simulink model "POMS_model_expanded"  (Simulink 7.9)
settings: Solver=VariableStepDiscrete  StartTime=0.0  StopTime=100.0  RelTol=1e-3
(part 2 of 2)

== system POMS_model_expanded/Depot_2/Storage_Subsystem/<<DELIVER>>Deliver_Stocked_Product/Deliver_Stocked_Product_CONTROL ==
  Calculate_Inventory_C : MATLAB Function  TreatAsAtomicUnit=on
  Combine_Consumption_Inventory : EntityCombiner  NumberInputPorts=2
  Consumption_Attributes : GetAttribute  AttributeName=Component|Consumption_Quantity|Net_Inventory|Inventory_Position  AttributeMissing=Error|Error|Error|Error  AttributeDefaultValue=1|1|1|1  AttributeTreatAsVector=1|1|1|1  AttributeSendTiming=After entity departure|After entity departure|After entity departure|After entity departure  EvaluatedDefaultAttributeValue={[];[];[];[]}
      settings: OutputPortMap=o1,o2,o3,o4
  Consumption_Server : SingleServer  ServiceTime=0
  Consumption_Sink : EntitySink
  Replicate : Replicate  NumberOutputPorts=2
  Return_Inventory : EntitySplitter  NumberOutputPorts=2
  Set_Inventory_Level : SetAttribute  AttributeName=Net_Inventory|Inventory_Position  AttributeFrom=Signal port|Signal port  AttributeValue=1|1  AttributeTreatAsVector=1|1  EvaluatedAttributeValue={[];[]}
      settings: InputPortMap=u0,u1
  Inventory_IN : PMIOPort  Port=1  Side=Left
  Consumption_Signal_IN : PMIOPort  Port=2  Side=Left
  Consumption_Signal_OUT : PMIOPort  Port=3  Side=Right
  Inventory_OUT : PMIOPort  Port=4  Side=Right
  wires:
  Calculate_Inventory_C/2(out_Inventory_Position) -> Set_Inventory_Level/2
  Consumption_Attributes/4 -> Calculate_Inventory_C/2(Inventory_Position)
  Consumption_Attributes/2 -> Calculate_Inventory_C/4(Consumption_Quantity)
  Consumption_Attributes/3 -> Calculate_Inventory_C/1(Net_Inventory)
  Calculate_Inventory_C/1(out_Net_Inventory) -> Set_Inventory_Level/1
  Consumption_Attributes/1 -> Calculate_Inventory_C/3(Component)
  connections:
  Consumption_Signal_IN/RConn1 -- Replicate/LConn1
  Inventory_OUT/RConn1 -- Return_Inventory/RConn1
  Set_Inventory_Level/RConn1 -- Return_Inventory/LConn1
  Replicate/RConn2 -- Consumption_Signal_OUT/RConn1
  Return_Inventory/RConn2 -- Consumption_Sink/LConn1
  Consumption_Server/RConn1 -- Set_Inventory_Level/LConn1
  Consumption_Attributes/RConn1 -- Consumption_Server/LConn1
  Combine_Consumption_Inventory/RConn1 -- Consumption_Attributes/LConn1
  Replicate/RConn1 -- Combine_Consumption_Inventory/LConn2
  Inventory_IN/RConn1 -- Combine_Consumption_Inventory/LConn1

== system POMS_model_expanded/Depot_2/Storage_Subsystem/<<DELIVER>>Deliver_Stocked_Product/sD1.10_Pack_Order_PLANT ==
  Entity Departure Function-Call Generator : EntityDepartureFunctionCallGenerator
  Event-Based Entity Generator : EventBasedEntityGenerator  GenerateEntitiesUpon=Function call from port fcn
  Get_Order_Attribute : GetAttribute  AttributeName=Component|Order_Quantity|Customer  AttributeMissing=Error|Error|Error  AttributeDefaultValue=1|1|1  AttributeTreatAsVector=1|1|1  AttributeSendTiming=After entity departure|After entity departure|After entity departure  EvaluatedDefaultAttributeValue={[];[];[]}
      settings: OutputPortMap=o1,o2,o3
  Order_Sink : EntitySink
  Set_Shipment_Attributes : SetAttribute  AttributeName=Component|Shipment_Quantity|Customer  AttributeFrom=Signal port|Signal port|Signal port  AttributeValue=1|1|1  AttributeTreatAsVector=1|1|1  EvaluatedAttributeValue={[];[];[]}
      settings: InputPortMap=u0,u1,u2
  sD1.10_Queue : FIFOQueue
  sD1.10_Server : NServer  NumberOfServers=inf  ServiceTime=0
  Order_IN : PMIOPort  Port=1  Side=Left
  Shipment_OUT : PMIOPort  Port=2  Side=Right
  wires:
  Get_Order_Attribute/3 -> Set_Shipment_Attributes/3
  Get_Order_Attribute/1 -> Set_Shipment_Attributes/1
  Get_Order_Attribute/2 -> Set_Shipment_Attributes/2
  Entity Departure Function-Call Generator/1 -> Event-Based Entity Generator/1
  connections:
  Get_Order_Attribute/RConn1 -- Entity Departure Function-Call Generator/LConn1
  sD1.10_Server/RConn1 -- Get_Order_Attribute/LConn1
  Order_Sink/LConn1 -- Entity Departure Function-Call Generator/RConn1
  Set_Shipment_Attributes/RConn1 -- Shipment_OUT/RConn1
  Event-Based Entity Generator/RConn1 -- Set_Shipment_Attributes/LConn1
  Order_IN/RConn1 -- sD1.10_Queue/LConn1
  sD1.10_Queue/RConn1 -- sD1.10_Server/LConn1

== system POMS_model_expanded/Depot_2/Storage_Subsystem/<<DELIVER>>Deliver_Stocked_Product/sD1.11_Load_Order_PLANT ==
  sD1.11_Queue : FIFOQueue
  sD1.11_Server : NServer  NumberOfServers=inf  ServiceTime=0
  Shipment_IN : PMIOPort  Port=1  Side=Left
  Shipment_OUT : PMIOPort  Port=2  Side=Right
  connections:
  Shipment_OUT/RConn1 -- sD1.11_Server/RConn1
  Shipment_IN/RConn1 -- sD1.11_Queue/LConn1
  sD1.11_Queue/RConn1 -- sD1.11_Server/LConn1

== system POMS_model_expanded/Depot_2/Storage_Subsystem/<<DELIVER>>Deliver_Stocked_Product/sD1.2_Receive_Order_PLANT ==
  sD1.2_Queue : FIFOQueue
  sD1.2_Server : NServer  NumberOfServers=inf  ServiceTime=0
  Order_IN : PMIOPort  Port=1  Side=Left
  Order_OUT : PMIOPort  Port=2  Side=Right
  connections:
  Order_OUT/RConn1 -- sD1.2_Server/RConn1
  Order_IN/RConn1 -- sD1.2_Queue/LConn1
  sD1.2_Queue/RConn1 -- sD1.2_Server/LConn1

== system POMS_model_expanded/Depot_2/Storage_Subsystem/<<DELIVER>>Deliver_Stocked_Product/sD1.4_Consolidate_Orders_PLANT ==
  sD1.4_Queue : FIFOQueue
  sD1.4_Server : NServer  NumberOfServers=inf  ServiceTime=0
  Order_IN : PMIOPort  Port=1  Side=Left
  Order_OUT : PMIOPort  Port=2  Side=Right
  connections:
  Order_OUT/RConn1 -- sD1.4_Server/RConn1
  Order_IN/RConn1 -- sD1.4_Queue/LConn1
  sD1.4_Queue/RConn1 -- sD1.4_Server/LConn1

== system POMS_model_expanded/Depot_2/Storage_Subsystem/<<DELIVER>>Deliver_Stocked_Product/sD1.9_Pick_Order_PLANT ==
  Generate_Consumption_Signal : Subsystem
  sD1.9_Queue : FIFOQueue
  sD1.9_Server : NServer  NumberOfServers=inf  ServiceTime=0
  Order_IN : PMIOPort  Port=1  Side=Left
  Consumption_Signal : PMIOPort  Port=2  Side=Right
  Order_OUT : PMIOPort  Port=3  Side=Right
  connections:
  Generate_Consumption_Signal/RConn2 -- Consumption_Signal/RConn1
  Generate_Consumption_Signal/RConn1 -- Order_OUT/RConn1
  sD1.9_Server/RConn1 -- Generate_Consumption_Signal/LConn1
  Order_IN/RConn1 -- sD1.9_Queue/LConn1
  sD1.9_Queue/RConn1 -- sD1.9_Server/LConn1

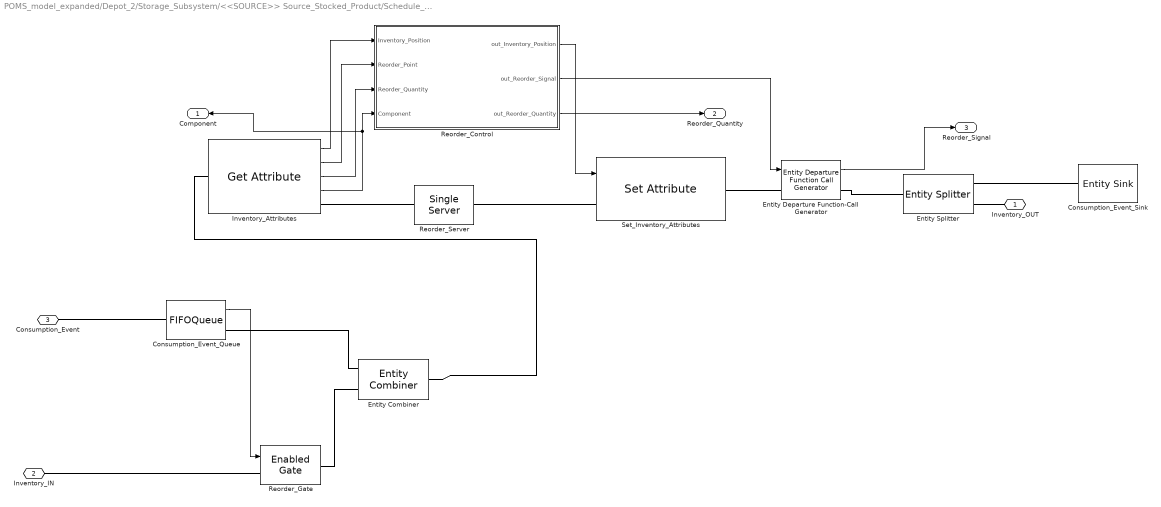
== system POMS_model_expanded/Depot_2/Storage_Subsystem/<<SOURCE>> Source_Stocked_Product/Schedule_Product_Deliveries_CONTROL ==
  Consumption_Event_Queue : FIFOQueue  StatNumberInBlock=on
      settings: OutputPortMap=o1
  Consumption_Event_Sink : EntitySink
  Entity Combiner : EntityCombiner  NumberInputPorts=2
  Entity Departure Function-Call Generator : EntityDepartureFunctionCallGenerator  EnableE1Port=on
  Entity Splitter : EntitySplitter  NumberOutputPorts=2
  Inventory_Attributes : GetAttribute  AttributeName=Inventory_Position|Reorder_Point|Reorder_Quantity|Component  AttributeMissing=Error|Error|Error|Error  AttributeDefaultValue=1|1|1|1  AttributeTreatAsVector=1|1|1|1  AttributeSendTiming=After entity departure|After entity departure|After entity departure|After entity departure  EvaluatedDefaultAttributeValue={[];[];[];[]}
      settings: OutputPortMap=o1,o2,o3,o4
  Reorder_Control : MATLAB Function  TreatAsAtomicUnit=on
  Reorder_Gate : EnabledGate
  Reorder_Server : SingleServer  ServiceTime=0
  Set_Inventory_Attributes : SetAttribute  AttributeName=Inventory_Position  AttributeFrom=Signal port  EvaluatedAttributeValue={[]}
  Inventory_OUT : PMIOPort  Port=1  Side=Right
  Inventory_IN : PMIOPort  Port=2  Side=Left
  Consumption_Event : PMIOPort  Port=3  Side=Left
  Component : Outport
  Reorder_Quantity : Outport  Port=2
  Reorder_Signal : Outport  Port=3
  wires:
  Entity Departure Function-Call Generator/1 -> Reorder_Signal/1
  Reorder_Control/3(out_Reorder_Quantity) -> Reorder_Quantity/1
  Consumption_Event_Queue/1 -> Reorder_Gate/1
  Reorder_Control/2(out_Reorder_Signal) -> Entity Departure Function-Call Generator/1
  Inventory_Attributes/4 -> Component/1, Reorder_Control/4(Component)
  Reorder_Control/1(out_Inventory_Position) -> Set_Inventory_Attributes/1
  Inventory_Attributes/3 -> Reorder_Control/3(Reorder_Quantity)
  Inventory_Attributes/2 -> Reorder_Control/2(Reorder_Point)
  Inventory_Attributes/1 -> Reorder_Control/1(Inventory_Position)
  connections:
  Entity Departure Function-Call Generator/RConn1 -- Entity Splitter/LConn1
  Set_Inventory_Attributes/RConn1 -- Entity Departure Function-Call Generator/LConn1
  Reorder_Server/RConn1 -- Set_Inventory_Attributes/LConn1
  Inventory_IN/RConn1 -- Reorder_Gate/LConn1
  Inventory_Attributes/RConn1 -- Reorder_Server/LConn1
  Inventory_OUT/RConn1 -- Entity Splitter/RConn2
  Entity Combiner/RConn1 -- Inventory_Attributes/LConn1
  Reorder_Gate/RConn1 -- Entity Combiner/LConn2
  Entity Splitter/RConn1 -- Consumption_Event_Sink/LConn1
  Consumption_Event_Queue/RConn1 -- Entity Combiner/LConn1
  Consumption_Event/RConn1 -- Consumption_Event_Queue/LConn1

== system POMS_model_expanded/Depot_2/Storage_Subsystem/<<SOURCE>> Source_Stocked_Product/Transfer_Product_CONTROL ==
  Calculate_Inventory : MATLAB Function  TreatAsAtomicUnit=on
  Combine_Inventory_and_Availability : EntityCombiner  NumberInputPorts=2
  FIFO Queue : FIFOQueue
  Inventory_Availability_Attributes : GetAttribute  AttributeName=Component|Shipment_Quantity|Net_Inventory  AttributeMissing=Error|Error|Error  AttributeDefaultValue=1|1|1  AttributeTreatAsVector=1|1|1  AttributeSendTiming=After entity departure|After entity departure|After entity departure  EvaluatedDefaultAttributeValue={[];[];[]}
      settings: OutputPortMap=o1,o2,o3
  Inventory_Availability_Sink : EntitySink
  Return_Inventory : EntitySplitter  NumberOutputPorts=2
  Server : SingleServer  ServiceTime=0
  Set_Inventory_Level : SetAttribute  AttributeName=Net_Inventory  AttributeFrom=Signal port  EvaluatedAttributeValue={[]}
  Inventory_OUT : PMIOPort  Port=1  Side=Right
  Inventory_IN : PMIOPort  Port=2  Side=Left
  Inventory_Availability_Signal : PMIOPort  Port=3  Side=Left
  wires:
  Inventory_Availability_Attributes/2 -> Calculate_Inventory/3(Shipment_Quantity)
  Inventory_Availability_Attributes/3 -> Calculate_Inventory/1(Net_Inventory)
  Calculate_Inventory/1(out_Inventory) -> Set_Inventory_Level/1
  Inventory_Availability_Attributes/1 -> Calculate_Inventory/2(Component)
  connections:
  Inventory_IN/RConn1 -- Combine_Inventory_and_Availability/LConn1
  FIFO Queue/RConn1 -- Combine_Inventory_and_Availability/LConn2
  Inventory_Availability_Signal/RConn1 -- FIFO Queue/LConn1
  Inventory_OUT/RConn1 -- Return_Inventory/RConn1
  Set_Inventory_Level/RConn1 -- Return_Inventory/LConn1
  Return_Inventory/RConn2 -- Inventory_Availability_Sink/LConn1
  Server/RConn1 -- Set_Inventory_Level/LConn1
  Inventory_Availability_Attributes/RConn1 -- Server/LConn1
  Combine_Inventory_and_Availability/RConn1 -- Inventory_Availability_Attributes/LConn1

== system POMS_model_expanded/Depot_2/Storage_Subsystem/<<SOURCE>> Source_Stocked_Product/sS1.1_Schedule_Product_Deliveries_PLANT ==
  Component : Inport
  Reorder_Quantity : Inport  Port=2
  Reorder_Signal : Inport  Port=3
  Generate_Procurement_Order : Subsystem
  Schedule_Product_Deliveries_Server : NServer  NumberOfServers=inf  ServiceTime=0
  Set_Procurement_Order : SetAttribute  AttributeName=Component|Order_Quantity|Supplier|Customer  AttributeFrom=Signal port|Signal port|Dialog|Dialog  AttributeValue=1|1|1|1  AttributeTreatAsVector=1|1|1|1  EvaluatedAttributeValue={[];[];1;1}
      settings: InputPortMap=u0,u1
  Procurement_Order : PMIOPort  Port=1  Side=Right
  wires:
  Reorder_Signal/1 -> Generate_Procurement_Order/1(Reorder_Signal)
  Reorder_Quantity/1 -> Set_Procurement_Order/2
  Component/1 -> Set_Procurement_Order/1
  connections:
  Procurement_Order/RConn1 -- Set_Procurement_Order/RConn1
  Schedule_Product_Deliveries_Server/RConn1 -- Set_Procurement_Order/LConn1
  Generate_Procurement_Order/RConn1 -- Schedule_Product_Deliveries_Server/LConn1

== system POMS_model_expanded/Depot_2/Storage_Subsystem/<<SOURCE>> Source_Stocked_Product/sS1.2_Receive_Product_PLANT ==
  sS1.2_Queue : FIFOQueue  Capacity=inf
  sS1.2_Server : NServer  NumberOfServers=inf  ServiceTime=0
  Shipment_IN : PMIOPort  Port=1  Side=Left
  Component_OUT : PMIOPort  Port=2  Side=Right
  connections:
  Component_OUT/RConn1 -- sS1.2_Server/RConn1
  Shipment_IN/RConn1 -- sS1.2_Queue/LConn1
  sS1.2_Queue/RConn1 -- sS1.2_Server/LConn1

== system POMS_model_expanded/Depot_2/Storage_Subsystem/<<SOURCE>> Source_Stocked_Product/sS1.3_Transfer_Product_PLANT ==
  sS1.4_Queue : FIFOQueue
  sS1.4_Server : NServer  NumberOfServers=inf  ServiceTime=0
  Component_IN : PMIOPort  Port=1  Side=Left
  Inventory_Availability_Signal : PMIOPort  Port=2  Side=Right
  connections:
  Inventory_Availability_Signal/RConn1 -- sS1.4_Server/RConn1
  Component_IN/RConn1 -- sS1.4_Queue/LConn1
  sS1.4_Queue/RConn1 -- sS1.4_Server/LConn1

== system POMS_model_expanded/Depot_2/Storage_Subsystem/<<SOURCE>> Source_Stocked_Product/sS1.3_Verify_Product_PLANT ==
  sS1.3_Queue : FIFOQueue  Capacity=inf
  sS1.3_Server : NServer  NumberOfServers=inf  ServiceTime=0
  Component_IN : PMIOPort  Port=1  Side=Left
  Component_OUT : PMIOPort  Port=2  Side=Right
  connections:
  Component_OUT/RConn1 -- sS1.3_Server/RConn1
  Component_IN/RConn1 -- sS1.3_Queue/LConn1
  sS1.3_Queue/RConn1 -- sS1.3_Server/LConn1

== system POMS_model_expanded/Hub_1/Storage_Subsystem/<<DELIVER>>Deliver_Stocked_Product/Deliver_Stocked_Product_CONTROL ==
  Calculate_Inventory_C : MATLAB Function  TreatAsAtomicUnit=on
  Combine_Consumption_Inventory : EntityCombiner  NumberInputPorts=2
  Consumption_Attributes : GetAttribute  AttributeName=Component|Consumption_Quantity|Net_Inventory|Inventory_Position  AttributeMissing=Error|Error|Error|Error  AttributeDefaultValue=1|1|1|1  AttributeTreatAsVector=1|1|1|1  AttributeSendTiming=After entity departure|After entity departure|After entity departure|After entity departure  EvaluatedDefaultAttributeValue={[];[];[];[]}
      settings: OutputPortMap=o1,o2,o3,o4
  Consumption_Server : SingleServer  ServiceTime=0
  Consumption_Sink : EntitySink
  Replicate : Replicate  NumberOutputPorts=2
  Return_Inventory : EntitySplitter  NumberOutputPorts=2
  Set_Inventory_Level : SetAttribute  AttributeName=Net_Inventory|Inventory_Position  AttributeFrom=Signal port|Signal port  AttributeValue=1|1  AttributeTreatAsVector=1|1  EvaluatedAttributeValue={[];[]}
      settings: InputPortMap=u0,u1
  Inventory_IN : PMIOPort  Port=1  Side=Left
  Consumption_Signal_IN : PMIOPort  Port=2  Side=Left
  Consumption_Signal_OUT : PMIOPort  Port=3  Side=Right
  Inventory_OUT : PMIOPort  Port=4  Side=Right
  wires:
  Calculate_Inventory_C/2(out_Inventory_Position) -> Set_Inventory_Level/2
  Consumption_Attributes/4 -> Calculate_Inventory_C/2(Inventory_Position)
  Consumption_Attributes/2 -> Calculate_Inventory_C/4(Consumption_Quantity)
  Consumption_Attributes/3 -> Calculate_Inventory_C/1(Net_Inventory)
  Calculate_Inventory_C/1(out_Net_Inventory) -> Set_Inventory_Level/1
  Consumption_Attributes/1 -> Calculate_Inventory_C/3(Component)
  connections:
  Consumption_Signal_IN/RConn1 -- Replicate/LConn1
  Inventory_OUT/RConn1 -- Return_Inventory/RConn1
  Set_Inventory_Level/RConn1 -- Return_Inventory/LConn1
  Replicate/RConn2 -- Consumption_Signal_OUT/RConn1
  Return_Inventory/RConn2 -- Consumption_Sink/LConn1
  Consumption_Server/RConn1 -- Set_Inventory_Level/LConn1
  Consumption_Attributes/RConn1 -- Consumption_Server/LConn1
  Combine_Consumption_Inventory/RConn1 -- Consumption_Attributes/LConn1
  Replicate/RConn1 -- Combine_Consumption_Inventory/LConn2
  Inventory_IN/RConn1 -- Combine_Consumption_Inventory/LConn1

== system POMS_model_expanded/Hub_1/Storage_Subsystem/<<DELIVER>>Deliver_Stocked_Product/sD1.10_Pack_Order_PLANT ==
  Entity Departure Function-Call Generator : EntityDepartureFunctionCallGenerator
  Event-Based Entity Generator : EventBasedEntityGenerator  GenerateEntitiesUpon=Function call from port fcn
  Get_Order_Attribute : GetAttribute  AttributeName=Component|Order_Quantity|Customer  AttributeMissing=Error|Error|Error  AttributeDefaultValue=1|1|1  AttributeTreatAsVector=1|1|1  AttributeSendTiming=After entity departure|After entity departure|After entity departure  EvaluatedDefaultAttributeValue={[];[];[]}
      settings: OutputPortMap=o1,o2,o3
  Order_Sink : EntitySink
  Set_Shipment_Attributes : SetAttribute  AttributeName=Component|Shipment_Quantity|Customer  AttributeFrom=Signal port|Signal port|Signal port  AttributeValue=1|1|1  AttributeTreatAsVector=1|1|1  EvaluatedAttributeValue={[];[];[]}
      settings: InputPortMap=u0,u1,u2
  sD1.10_Queue : FIFOQueue
  sD1.10_Server : NServer  NumberOfServers=inf  ServiceTime=0
  Order_IN : PMIOPort  Port=1  Side=Left
  Shipment_OUT : PMIOPort  Port=2  Side=Right
  wires:
  Get_Order_Attribute/3 -> Set_Shipment_Attributes/3
  Get_Order_Attribute/1 -> Set_Shipment_Attributes/1
  Get_Order_Attribute/2 -> Set_Shipment_Attributes/2
  Entity Departure Function-Call Generator/1 -> Event-Based Entity Generator/1
  connections:
  Get_Order_Attribute/RConn1 -- Entity Departure Function-Call Generator/LConn1
  sD1.10_Server/RConn1 -- Get_Order_Attribute/LConn1
  Order_Sink/LConn1 -- Entity Departure Function-Call Generator/RConn1
  Set_Shipment_Attributes/RConn1 -- Shipment_OUT/RConn1
  Event-Based Entity Generator/RConn1 -- Set_Shipment_Attributes/LConn1
  Order_IN/RConn1 -- sD1.10_Queue/LConn1
  sD1.10_Queue/RConn1 -- sD1.10_Server/LConn1

== system POMS_model_expanded/Hub_1/Storage_Subsystem/<<DELIVER>>Deliver_Stocked_Product/sD1.11_Load_Order_PLANT ==
  sD1.11_Queue : FIFOQueue
  sD1.11_Server : NServer  NumberOfServers=inf  ServiceTime=0
  Shipment_IN : PMIOPort  Port=1  Side=Left
  Shipment_OUT : PMIOPort  Port=2  Side=Right
  connections:
  Shipment_OUT/RConn1 -- sD1.11_Server/RConn1
  Shipment_IN/RConn1 -- sD1.11_Queue/LConn1
  sD1.11_Queue/RConn1 -- sD1.11_Server/LConn1

== system POMS_model_expanded/Hub_1/Storage_Subsystem/<<DELIVER>>Deliver_Stocked_Product/sD1.2_Receive_Order_PLANT ==
  sD1.2_Queue : FIFOQueue
  sD1.2_Server : NServer  NumberOfServers=inf  ServiceTime=0
  Order_IN : PMIOPort  Port=1  Side=Left
  Order_OUT : PMIOPort  Port=2  Side=Right
  connections:
  Order_OUT/RConn1 -- sD1.2_Server/RConn1
  Order_IN/RConn1 -- sD1.2_Queue/LConn1
  sD1.2_Queue/RConn1 -- sD1.2_Server/LConn1

== system POMS_model_expanded/Hub_1/Storage_Subsystem/<<DELIVER>>Deliver_Stocked_Product/sD1.4_Consolidate_Orders_PLANT ==
  sD1.4_Queue : FIFOQueue
  sD1.4_Server : NServer  NumberOfServers=inf  ServiceTime=0
  Order_IN : PMIOPort  Port=1  Side=Left
  Order_OUT : PMIOPort  Port=2  Side=Right
  connections:
  Order_OUT/RConn1 -- sD1.4_Server/RConn1
  Order_IN/RConn1 -- sD1.4_Queue/LConn1
  sD1.4_Queue/RConn1 -- sD1.4_Server/LConn1

== system POMS_model_expanded/Hub_1/Storage_Subsystem/<<DELIVER>>Deliver_Stocked_Product/sD1.9_Pick_Order_PLANT ==
  Generate_Consumption_Signal : Subsystem
  sD1.9_Queue : FIFOQueue
  sD1.9_Server : NServer  NumberOfServers=inf  ServiceTime=0
  Order_IN : PMIOPort  Port=1  Side=Left
  Consumption_Signal : PMIOPort  Port=2  Side=Right
  Order_OUT : PMIOPort  Port=3  Side=Right
  connections:
  Generate_Consumption_Signal/RConn2 -- Consumption_Signal/RConn1
  Generate_Consumption_Signal/RConn1 -- Order_OUT/RConn1
  sD1.9_Server/RConn1 -- Generate_Consumption_Signal/LConn1
  Order_IN/RConn1 -- sD1.9_Queue/LConn1
  sD1.9_Queue/RConn1 -- sD1.9_Server/LConn1

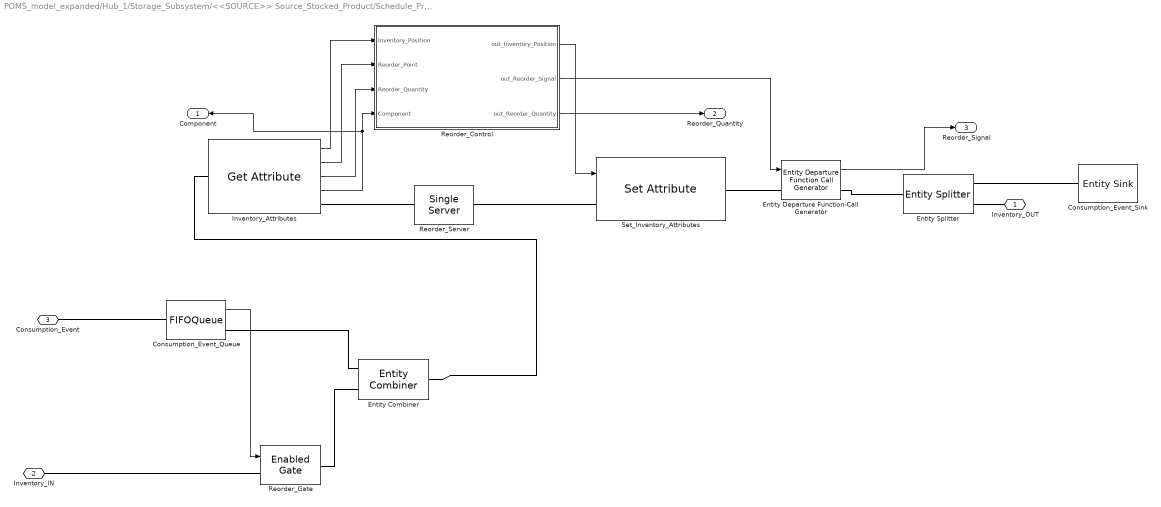
== system POMS_model_expanded/Hub_1/Storage_Subsystem/<<SOURCE>> Source_Stocked_Product/Schedule_Product_Deliveries_CONTROL ==
  Consumption_Event_Queue : FIFOQueue  StatNumberInBlock=on
      settings: OutputPortMap=o1
  Consumption_Event_Sink : EntitySink
  Entity Combiner : EntityCombiner  NumberInputPorts=2
  Entity Departure Function-Call Generator : EntityDepartureFunctionCallGenerator  EnableE1Port=on
  Entity Splitter : EntitySplitter  NumberOutputPorts=2
  Inventory_Attributes : GetAttribute  AttributeName=Inventory_Position|Reorder_Point|Reorder_Quantity|Component  AttributeMissing=Error|Error|Error|Error  AttributeDefaultValue=1|1|1|1  AttributeTreatAsVector=1|1|1|1  AttributeSendTiming=After entity departure|After entity departure|After entity departure|After entity departure  EvaluatedDefaultAttributeValue={[];[];[];[]}
      settings: OutputPortMap=o1,o2,o3,o4
  Reorder_Control : MATLAB Function  TreatAsAtomicUnit=on
  Reorder_Gate : EnabledGate
  Reorder_Server : SingleServer  ServiceTime=0
  Set_Inventory_Attributes : SetAttribute  AttributeName=Inventory_Position  AttributeFrom=Signal port  EvaluatedAttributeValue={[]}
  Inventory_OUT : PMIOPort  Port=1  Side=Right
  Inventory_IN : PMIOPort  Port=2  Side=Left
  Consumption_Event : PMIOPort  Port=3  Side=Left
  Component : Outport
  Reorder_Quantity : Outport  Port=2
  Reorder_Signal : Outport  Port=3
  wires:
  Entity Departure Function-Call Generator/1 -> Reorder_Signal/1
  Reorder_Control/3(out_Reorder_Quantity) -> Reorder_Quantity/1
  Consumption_Event_Queue/1 -> Reorder_Gate/1
  Reorder_Control/2(out_Reorder_Signal) -> Entity Departure Function-Call Generator/1
  Inventory_Attributes/4 -> Component/1, Reorder_Control/4(Component)
  Reorder_Control/1(out_Inventory_Position) -> Set_Inventory_Attributes/1
  Inventory_Attributes/3 -> Reorder_Control/3(Reorder_Quantity)
  Inventory_Attributes/2 -> Reorder_Control/2(Reorder_Point)
  Inventory_Attributes/1 -> Reorder_Control/1(Inventory_Position)
  connections:
  Entity Departure Function-Call Generator/RConn1 -- Entity Splitter/LConn1
  Set_Inventory_Attributes/RConn1 -- Entity Departure Function-Call Generator/LConn1
  Reorder_Server/RConn1 -- Set_Inventory_Attributes/LConn1
  Inventory_IN/RConn1 -- Reorder_Gate/LConn1
  Inventory_Attributes/RConn1 -- Reorder_Server/LConn1
  Inventory_OUT/RConn1 -- Entity Splitter/RConn2
  Entity Combiner/RConn1 -- Inventory_Attributes/LConn1
  Reorder_Gate/RConn1 -- Entity Combiner/LConn2
  Entity Splitter/RConn1 -- Consumption_Event_Sink/LConn1
  Consumption_Event_Queue/RConn1 -- Entity Combiner/LConn1
  Consumption_Event/RConn1 -- Consumption_Event_Queue/LConn1

== system POMS_model_expanded/Hub_1/Storage_Subsystem/<<SOURCE>> Source_Stocked_Product/Transfer_Product_CONTROL ==
  Calculate_Inventory : MATLAB Function  TreatAsAtomicUnit=on
  Combine_Inventory_and_Availability : EntityCombiner  NumberInputPorts=2
  FIFO Queue : FIFOQueue
  Inventory_Availability_Attributes : GetAttribute  AttributeName=Component|Shipment_Quantity|Net_Inventory  AttributeMissing=Error|Error|Error  AttributeDefaultValue=1|1|1  AttributeTreatAsVector=1|1|1  AttributeSendTiming=After entity departure|After entity departure|After entity departure  EvaluatedDefaultAttributeValue={[];[];[]}
      settings: OutputPortMap=o1,o2,o3
  Inventory_Availability_Sink : EntitySink
  Return_Inventory : EntitySplitter  NumberOutputPorts=2
  Server : SingleServer  ServiceTime=0
  Set_Inventory_Level : SetAttribute  AttributeName=Net_Inventory  AttributeFrom=Signal port  EvaluatedAttributeValue={[]}
  Inventory_OUT : PMIOPort  Port=1  Side=Right
  Inventory_IN : PMIOPort  Port=2  Side=Left
  Inventory_Availability_Signal : PMIOPort  Port=3  Side=Left
  wires:
  Inventory_Availability_Attributes/2 -> Calculate_Inventory/3(Shipment_Quantity)
  Inventory_Availability_Attributes/3 -> Calculate_Inventory/1(Net_Inventory)
  Calculate_Inventory/1(out_Inventory) -> Set_Inventory_Level/1
  Inventory_Availability_Attributes/1 -> Calculate_Inventory/2(Component)
  connections:
  Inventory_IN/RConn1 -- Combine_Inventory_and_Availability/LConn1
  FIFO Queue/RConn1 -- Combine_Inventory_and_Availability/LConn2
  Inventory_Availability_Signal/RConn1 -- FIFO Queue/LConn1
  Inventory_OUT/RConn1 -- Return_Inventory/RConn1
  Set_Inventory_Level/RConn1 -- Return_Inventory/LConn1
  Return_Inventory/RConn2 -- Inventory_Availability_Sink/LConn1
  Server/RConn1 -- Set_Inventory_Level/LConn1
  Inventory_Availability_Attributes/RConn1 -- Server/LConn1
  Combine_Inventory_and_Availability/RConn1 -- Inventory_Availability_Attributes/LConn1

== system POMS_model_expanded/Hub_1/Storage_Subsystem/<<SOURCE>> Source_Stocked_Product/sS1.1_Schedule_Product_Deliveries_PLANT ==
  Component : Inport
  Reorder_Quantity : Inport  Port=2
  Reorder_Signal : Inport  Port=3
  Generate_Procurement_Order : Subsystem
  Schedule_Product_Deliveries_Server : NServer  NumberOfServers=inf  ServiceTime=0
  Set_Procurement_Order : SetAttribute  AttributeName=Component|Order_Quantity|Supplier|Customer  AttributeFrom=Signal port|Signal port|Dialog|Dialog  AttributeValue=1|1|1|1  AttributeTreatAsVector=1|1|1|1  EvaluatedAttributeValue={[];[];1;1}
      settings: InputPortMap=u0,u1
  Procurement_Order : PMIOPort  Port=1  Side=Right
  wires:
  Reorder_Signal/1 -> Generate_Procurement_Order/1(Reorder_Signal)
  Reorder_Quantity/1 -> Set_Procurement_Order/2
  Component/1 -> Set_Procurement_Order/1
  connections:
  Procurement_Order/RConn1 -- Set_Procurement_Order/RConn1
  Schedule_Product_Deliveries_Server/RConn1 -- Set_Procurement_Order/LConn1
  Generate_Procurement_Order/RConn1 -- Schedule_Product_Deliveries_Server/LConn1

== system POMS_model_expanded/Hub_1/Storage_Subsystem/<<SOURCE>> Source_Stocked_Product/sS1.2_Receive_Product_PLANT ==
  sS1.2_Queue : FIFOQueue  Capacity=inf
  sS1.2_Server : NServer  NumberOfServers=inf  ServiceTime=0
  Shipment_IN : PMIOPort  Port=1  Side=Left
  Component_OUT : PMIOPort  Port=2  Side=Right
  connections:
  Component_OUT/RConn1 -- sS1.2_Server/RConn1
  Shipment_IN/RConn1 -- sS1.2_Queue/LConn1
  sS1.2_Queue/RConn1 -- sS1.2_Server/LConn1

== system POMS_model_expanded/Hub_1/Storage_Subsystem/<<SOURCE>> Source_Stocked_Product/sS1.3_Transfer_Product_PLANT ==
  sS1.4_Queue : FIFOQueue
  sS1.4_Server : NServer  NumberOfServers=inf  ServiceTime=0
  Component_IN : PMIOPort  Port=1  Side=Left
  Inventory_Availability_Signal : PMIOPort  Port=2  Side=Right
  connections:
  Inventory_Availability_Signal/RConn1 -- sS1.4_Server/RConn1
  Component_IN/RConn1 -- sS1.4_Queue/LConn1
  sS1.4_Queue/RConn1 -- sS1.4_Server/LConn1

== system POMS_model_expanded/Hub_1/Storage_Subsystem/<<SOURCE>> Source_Stocked_Product/sS1.3_Verify_Product_PLANT ==
  sS1.3_Queue : FIFOQueue  Capacity=inf
  sS1.3_Server : NServer  NumberOfServers=inf  ServiceTime=0
  Component_IN : PMIOPort  Port=1  Side=Left
  Component_OUT : PMIOPort  Port=2  Side=Right
  connections:
  Component_OUT/RConn1 -- sS1.3_Server/RConn1
  Component_IN/RConn1 -- sS1.3_Queue/LConn1
  sS1.3_Queue/RConn1 -- sS1.3_Server/LConn1

== system POMS_model_expanded/Depot_1/Storage_Subsystem/<<DELIVER>>Deliver_Stocked_Product/sD1.9_Pick_Order_PLANT/Generate_Consumption_Signal ==
  Entity Departure Function-Call Generator : EntityDepartureFunctionCallGenerator
  Event-Based Entity Generator : EventBasedEntityGenerator  GenerateEntitiesUpon=Function call from port fcn
  Get_Order_Attributes : GetAttribute  AttributeName=Component|Order_Quantity  AttributeMissing=Error|Error  AttributeDefaultValue=1|1  AttributeTreatAsVector=1|1  AttributeSendTiming=After entity departure|After entity departure  EvaluatedDefaultAttributeValue={[];[]}
      settings: OutputPortMap=o1,o2
  Set_Consumption_Attributes : SetAttribute  AttributeName=Component|Consumption_Quantity  AttributeFrom=Signal port|Signal port  AttributeValue=1|1  AttributeTreatAsVector=1|1  EvaluatedAttributeValue={[];[]}
      settings: InputPortMap=u0,u1
  Order_IN : PMIOPort  Port=1  Side=Left
  Order_OUT : PMIOPort  Port=2  Side=Right
  Consumption_Signal : PMIOPort  Port=3  Side=Right
  wires:
  Get_Order_Attributes/2 -> Set_Consumption_Attributes/2
  Get_Order_Attributes/1 -> Set_Consumption_Attributes/1
  Entity Departure Function-Call Generator/1 -> Event-Based Entity Generator/1
  connections:
  Order_IN/RConn1 -- Get_Order_Attributes/LConn1
  Set_Consumption_Attributes/RConn1 -- Consumption_Signal/RConn1
  Event-Based Entity Generator/RConn1 -- Set_Consumption_Attributes/LConn1
  Entity Departure Function-Call Generator/RConn1 -- Order_OUT/RConn1
  Get_Order_Attributes/RConn1 -- Entity Departure Function-Call Generator/LConn1

== system POMS_model_expanded/Depot_1/Storage_Subsystem/<<SOURCE>> Source_Stocked_Product/sS1.1_Schedule_Product_Deliveries_PLANT/Generate_Procurement_Order ==
  Reorder_Signal : Inport
  Event-Based Entity Generator : EventBasedEntityGenerator  GenerateEntitiesUpon=Function call from port fcn
  Blank_Procurement_Order : PMIOPort  Port=1  Side=Right
  wires:
  Reorder_Signal/1 -> Event-Based Entity Generator/1
  connections:
  Blank_Procurement_Order/RConn1 -- Event-Based Entity Generator/RConn1

== system POMS_model_expanded/Depot_2/Storage_Subsystem/<<DELIVER>>Deliver_Stocked_Product/sD1.9_Pick_Order_PLANT/Generate_Consumption_Signal ==
  Entity Departure Function-Call Generator : EntityDepartureFunctionCallGenerator
  Event-Based Entity Generator : EventBasedEntityGenerator  GenerateEntitiesUpon=Function call from port fcn
  Get_Order_Attributes : GetAttribute  AttributeName=Component|Order_Quantity  AttributeMissing=Error|Error  AttributeDefaultValue=1|1  AttributeTreatAsVector=1|1  AttributeSendTiming=After entity departure|After entity departure  EvaluatedDefaultAttributeValue={[];[]}
      settings: OutputPortMap=o1,o2
  Set_Consumption_Attributes : SetAttribute  AttributeName=Component|Consumption_Quantity  AttributeFrom=Signal port|Signal port  AttributeValue=1|1  AttributeTreatAsVector=1|1  EvaluatedAttributeValue={[];[]}
      settings: InputPortMap=u0,u1
  Order_IN : PMIOPort  Port=1  Side=Left
  Order_OUT : PMIOPort  Port=2  Side=Right
  Consumption_Signal : PMIOPort  Port=3  Side=Right
  wires:
  Get_Order_Attributes/2 -> Set_Consumption_Attributes/2
  Get_Order_Attributes/1 -> Set_Consumption_Attributes/1
  Entity Departure Function-Call Generator/1 -> Event-Based Entity Generator/1
  connections:
  Order_IN/RConn1 -- Get_Order_Attributes/LConn1
  Set_Consumption_Attributes/RConn1 -- Consumption_Signal/RConn1
  Event-Based Entity Generator/RConn1 -- Set_Consumption_Attributes/LConn1
  Entity Departure Function-Call Generator/RConn1 -- Order_OUT/RConn1
  Get_Order_Attributes/RConn1 -- Entity Departure Function-Call Generator/LConn1

== system POMS_model_expanded/Depot_2/Storage_Subsystem/<<SOURCE>> Source_Stocked_Product/sS1.1_Schedule_Product_Deliveries_PLANT/Generate_Procurement_Order ==
  Reorder_Signal : Inport
  Event-Based Entity Generator : EventBasedEntityGenerator  GenerateEntitiesUpon=Function call from port fcn
  Blank_Procurement_Order : PMIOPort  Port=1  Side=Right
  wires:
  Reorder_Signal/1 -> Event-Based Entity Generator/1
  connections:
  Blank_Procurement_Order/RConn1 -- Event-Based Entity Generator/RConn1

== system POMS_model_expanded/Hub_1/Storage_Subsystem/<<DELIVER>>Deliver_Stocked_Product/sD1.9_Pick_Order_PLANT/Generate_Consumption_Signal ==
  Entity Departure Function-Call Generator : EntityDepartureFunctionCallGenerator
  Event-Based Entity Generator : EventBasedEntityGenerator  GenerateEntitiesUpon=Function call from port fcn
  Get_Order_Attributes : GetAttribute  AttributeName=Component|Order_Quantity  AttributeMissing=Error|Error  AttributeDefaultValue=1|1  AttributeTreatAsVector=1|1  AttributeSendTiming=After entity departure|After entity departure  EvaluatedDefaultAttributeValue={[];[]}
      settings: OutputPortMap=o1,o2
  Set_Consumption_Attributes : SetAttribute  AttributeName=Component|Consumption_Quantity  AttributeFrom=Signal port|Signal port  AttributeValue=1|1  AttributeTreatAsVector=1|1  EvaluatedAttributeValue={[];[]}
      settings: InputPortMap=u0,u1
  Order_IN : PMIOPort  Port=1  Side=Left
  Order_OUT : PMIOPort  Port=2  Side=Right
  Consumption_Signal : PMIOPort  Port=3  Side=Right
  wires:
  Get_Order_Attributes/2 -> Set_Consumption_Attributes/2
  Get_Order_Attributes/1 -> Set_Consumption_Attributes/1
  Entity Departure Function-Call Generator/1 -> Event-Based Entity Generator/1
  connections:
  Order_IN/RConn1 -- Get_Order_Attributes/LConn1
  Set_Consumption_Attributes/RConn1 -- Consumption_Signal/RConn1
  Event-Based Entity Generator/RConn1 -- Set_Consumption_Attributes/LConn1
  Entity Departure Function-Call Generator/RConn1 -- Order_OUT/RConn1
  Get_Order_Attributes/RConn1 -- Entity Departure Function-Call Generator/LConn1

== system POMS_model_expanded/Hub_1/Storage_Subsystem/<<SOURCE>> Source_Stocked_Product/sS1.1_Schedule_Product_Deliveries_PLANT/Generate_Procurement_Order ==
  Reorder_Signal : Inport
  Event-Based Entity Generator : EventBasedEntityGenerator  GenerateEntitiesUpon=Function call from port fcn
  Blank_Procurement_Order : PMIOPort  Port=1  Side=Right
  wires:
  Reorder_Signal/1 -> Event-Based Entity Generator/1
  connections:
  Blank_Procurement_Order/RConn1 -- Event-Based Entity Generator/RConn1

== matlab function Hub_1/Storage_Subsystem/<<DELIVER>>Deliver_Stocked_Product/Deliver_Stocked_Product_CONTROL/Calculate_Inventory_C ==
  data: Net_Inventory input double; Inventory_Position input double; out_Net_Inventory output double; Component input double; Consumption_Quantity input double; out_Inventory_Position output double
function [out_Net_Inventory,out_Inventory_Position] = fcn(Net_Inventory, Inventory_Position, Component, Consumption_Quantity)
%#codegen

%coder.extrinsic('str2num');

%y = zeros(1, 'int32');
%y = Type;
out_Net_Inventory = Net_Inventory;
out_Inventory_Position = Inventory_Position;
if eq(Component, 0) == 0
    out_Net_Inventory(Component) = Net_Inventory(Component) - Consumption_Quantity;
    out_Inventory_Position(Component) = Inventory_Position(Component) - Consumption_Quantity;
end

end

== matlab function Hub_1/Storage_Subsystem/<<SOURCE>> Source_Stocked_Product/Schedule_Product_Deliveries_CONTROL/Reorder_Control ==
  data: Inventory_Position input double; Reorder_Point input double; Reorder_Quantity input double; Component input double; out_Inventory_Position output double; out_Reorder_Signal output double; out_Reorder_Quantity output double
function [out_Inventory_Position, out_Reorder_Signal, out_Reorder_Quantity] = fcn(Inventory_Position, Reorder_Point, Reorder_Quantity, Component)
%This function is a combination of all the CONTROL systems at once

out_Inventory_Position = Inventory_Position;
out_Reorder_Signal =0;
out_Reorder_Quantity = 0;
if eq(Component, 0) == 0
    %Operative Subsystem Control
    if Inventory_Position(Component) <= Reorder_Point(Component)
        out_Reorder_Signal = Reorder_Quantity(Component);
        out_Reorder_Quantity = Reorder_Quantity(Component);
        
        %Control & Monitoring Subsystem
        out_Inventory_Position(Component) = Inventory_Position(Component) + Reorder_Quantity(Component);
        
    end
end

== matlab function Hub_1/Storage_Subsystem/<<SOURCE>> Source_Stocked_Product/Transfer_Product_CONTROL/Calculate_Inventory ==
  data: Net_Inventory input double; out_Inventory output double; Component input double; Shipment_Quantity input double
function out_Inventory = fcn(Net_Inventory, Component, Shipment_Quantity)
%#codegen

%coder.extrinsic('str2num');

%y = zeros(1, 'int32');
%y = Type;
out_Inventory = Net_Inventory;
if eq(Component, 0) == 0
    out_Inventory(Component) = Net_Inventory(Component) + Shipment_Quantity;
end

end

== matlab function Depot_1/Storage_Subsystem/<<DELIVER>>Deliver_Stocked_Product/Deliver_Stocked_Product_CONTROL/Calculate_Inventory_C ==
  data: Net_Inventory input double; Inventory_Position input double; out_Net_Inventory output double; Component input double; Consumption_Quantity input double; out_Inventory_Position output double
function [out_Net_Inventory,out_Inventory_Position] = fcn(Net_Inventory, Inventory_Position, Component, Consumption_Quantity)
%#codegen

%coder.extrinsic('str2num');

%y = zeros(1, 'int32');
%y = Type;
out_Net_Inventory = Net_Inventory;
out_Inventory_Position = Inventory_Position;
if eq(Component, 0) == 0
    out_Net_Inventory(Component) = Net_Inventory(Component) - Consumption_Quantity;
    out_Inventory_Position(Component) = Inventory_Position(Component) - Consumption_Quantity;
end

end

== matlab function Depot_1/Storage_Subsystem/<<SOURCE>> Source_Stocked_Product/Schedule_Product_Deliveries_CONTROL/Reorder_Control ==
  data: Inventory_Position input double; Reorder_Point input double; Reorder_Quantity input double; Component input double; out_Inventory_Position output double; out_Reorder_Signal output double; out_Reorder_Quantity output double
function [out_Inventory_Position, out_Reorder_Signal, out_Reorder_Quantity] = fcn(Inventory_Position, Reorder_Point, Reorder_Quantity, Component)
%This function is a combination of all the CONTROL systems at once

out_Inventory_Position = Inventory_Position;
out_Reorder_Signal =0;
out_Reorder_Quantity = 0;
if eq(Component, 0) == 0
    %Operative Subsystem Control
    if Inventory_Position(Component) <= Reorder_Point(Component)
        out_Reorder_Signal = Reorder_Quantity(Component);
        out_Reorder_Quantity = Reorder_Quantity(Component);
        
        %Control & Monitoring Subsystem
        out_Inventory_Position(Component) = Inventory_Position(Component) + Reorder_Quantity(Component);
        
    end
end

== matlab function Depot_1/Storage_Subsystem/<<SOURCE>> Source_Stocked_Product/Transfer_Product_CONTROL/Calculate_Inventory ==
  data: Net_Inventory input double; out_Inventory output double; Component input double; Shipment_Quantity input double
function out_Inventory = fcn(Net_Inventory, Component, Shipment_Quantity)
%#codegen

%coder.extrinsic('str2num');

%y = zeros(1, 'int32');
%y = Type;
out_Inventory = Net_Inventory;
if eq(Component, 0) == 0
    out_Inventory(Component) = Net_Inventory(Component) + Shipment_Quantity;
end

end

== matlab function Depot_2/Storage_Subsystem/<<DELIVER>>Deliver_Stocked_Product/Deliver_Stocked_Product_CONTROL/Calculate_Inventory_C ==
  data: Net_Inventory input double; Inventory_Position input double; out_Net_Inventory output double; Component input double; Consumption_Quantity input double; out_Inventory_Position output double
function [out_Net_Inventory,out_Inventory_Position] = fcn(Net_Inventory, Inventory_Position, Component, Consumption_Quantity)
%#codegen

%coder.extrinsic('str2num');

%y = zeros(1, 'int32');
%y = Type;
out_Net_Inventory = Net_Inventory;
out_Inventory_Position = Inventory_Position;
if eq(Component, 0) == 0
    out_Net_Inventory(Component) = Net_Inventory(Component) - Consumption_Quantity;
    out_Inventory_Position(Component) = Inventory_Position(Component) - Consumption_Quantity;
end

end

== matlab function Depot_2/Storage_Subsystem/<<SOURCE>> Source_Stocked_Product/Schedule_Product_Deliveries_CONTROL/Reorder_Control ==
  data: Inventory_Position input double; Reorder_Point input double; Reorder_Quantity input double; Component input double; out_Inventory_Position output double; out_Reorder_Signal output double; out_Reorder_Quantity output double
function [out_Inventory_Position, out_Reorder_Signal, out_Reorder_Quantity] = fcn(Inventory_Position, Reorder_Point, Reorder_Quantity, Component)
%This function is a combination of all the CONTROL systems at once

out_Inventory_Position = Inventory_Position;
out_Reorder_Signal =0;
out_Reorder_Quantity = 0;
if eq(Component, 0) == 0
    %Operative Subsystem Control
    if Inventory_Position(Component) <= Reorder_Point(Component)
        out_Reorder_Signal = Reorder_Quantity(Component);
        out_Reorder_Quantity = Reorder_Quantity(Component);
        
        %Control & Monitoring Subsystem
        out_Inventory_Position(Component) = Inventory_Position(Component) + Reorder_Quantity(Component);
        
    end
end

== matlab function Depot_2/Storage_Subsystem/<<SOURCE>> Source_Stocked_Product/Transfer_Product_CONTROL/Calculate_Inventory ==
  data: Net_Inventory input double; out_Inventory output double; Component input double; Shipment_Quantity input double
function out_Inventory = fcn(Net_Inventory, Component, Shipment_Quantity)
%#codegen

%coder.extrinsic('str2num');

%y = zeros(1, 'int32');
%y = Type;
out_Inventory = Net_Inventory;
if eq(Component, 0) == 0
    out_Inventory(Component) = Net_Inventory(Component) + Shipment_Quantity;
end

end
